simulink model "msdTune"  (R2022b)
settings: Solver=ode23t  StartTime=0.0  StopTime=10  MaxStep=1e-5  RelTol=1e-6
libraries: simulink x2
settings Model: Creator=Rocksmithed  LastModifiedBy=86156
settings SolverCC: AlgebraicLoopSolver=TrustRegion
settings DebuggingCC: UnconnectedInputMsg=warning  UnconnectedOutputMsg=warning  UnconnectedLineMsg=warning  SFMachineParentedDataDiag=warning
settings ModelReferenceCC: EnableRefExpFcnMdlSchedulingChecks=on
settings RTWCC: DLArmComputeVersion=19.05

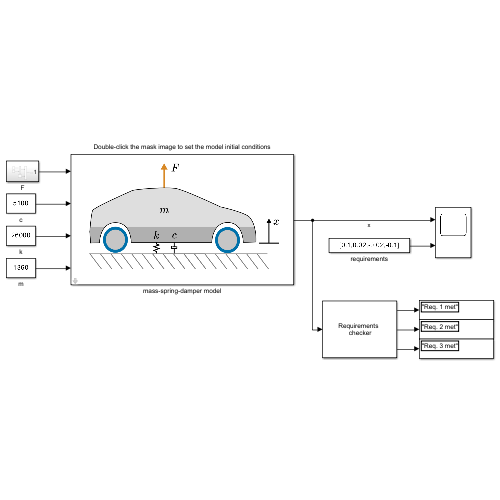
[thumbnail: Simulink's stored preview of the top-level diagram]
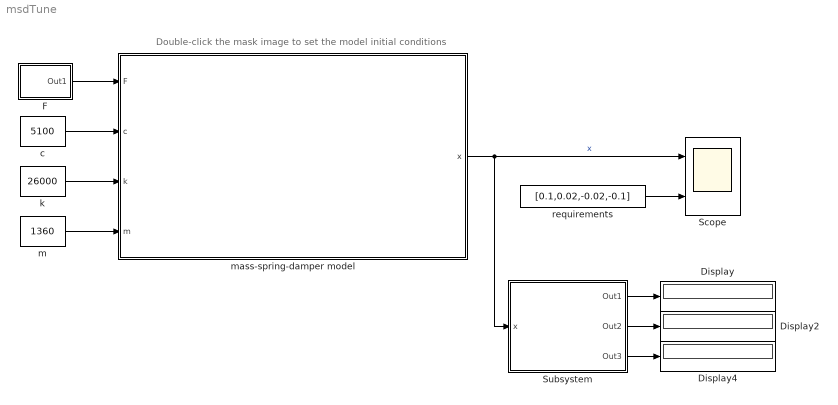
== system msdTune ==
  note: Double-click the mask image to set the model initial conditions
  Display : Display
  Display2 : Display
  Display4 : Display
  F : Subsystem
  Scope : Scope  NumInputPorts=2
  Subsystem : Subsystem
      mask Display: disp('Requirements \n checker')
  c : Constant  Value=5100
  k : Constant  Value=26000
  m : Constant  Value=1360
  mass-spring-damper model : Subsystem  mask{x0=0, x_dot0=0}
      mask prompts: x_dot0 "x'(0)"
      mask Display: image('$imagefile'); % Use "Edit Image" on toolstrip to change.
  requirements : Constant  Value=[0.1,0.02,-0.02,-0.1]
  wires:
  c/1 -> mass-spring-damper model/2(c)
  k/1 -> mass-spring-damper model/3(k)
  m/1 -> mass-spring-damper model/4(m)
  mass-spring-damper model/1(x) -> Subsystem/1(x), Scope/1  "x"
  F/1(Out1) -> mass-spring-damper model/1(F)
  requirements/1 -> Scope/2
  Subsystem/1(Out1) -> Display/1
  Subsystem/2(Out2) -> Display2/1
  Subsystem/3(Out3) -> Display4/1

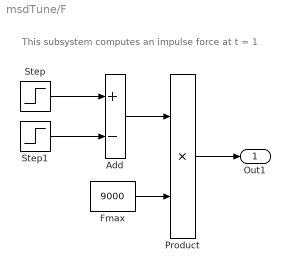
== system msdTune/F ==
  note: This subsystem computes an impulse force at t = 1
  Add : Sum  Inputs=+-
  Fmax : Constant  Value=9000
  Product : Product
  Step : Step  SampleTime=0
  Step1 : Step  Time=1.1  SampleTime=0
  Out1 : Outport
  wires:
  Product/1 -> Out1/1
  Add/1 -> Product/1
  Fmax/1 -> Product/2
  Step/1 -> Add/1
  Step1/1 -> Add/2

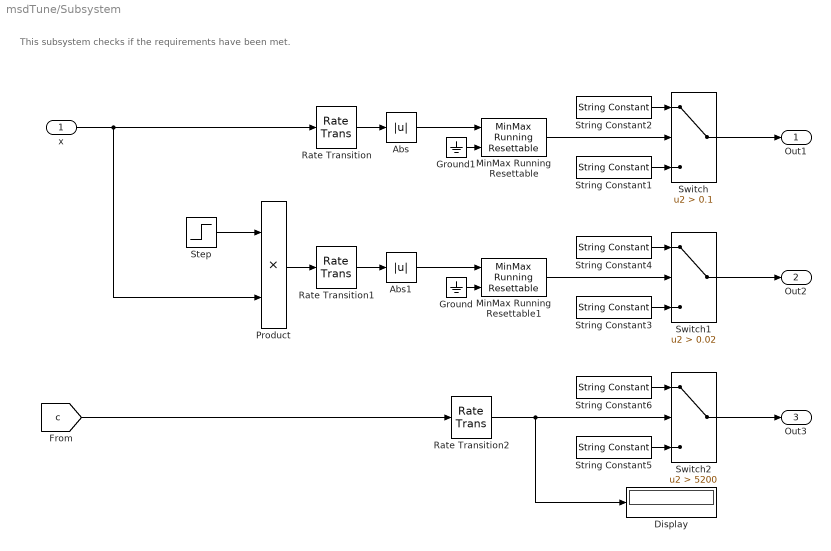
== system msdTune/Subsystem ==
  note: This subsystem checks if the requirements have been met.
  x : Inport
  Abs : Abs  SaturateOnIntegerOverflow=off
  Abs1 : Abs  SaturateOnIntegerOverflow=off
  Display : Display
  Ground : Ground
  Ground1 : Ground
  MinMax Running Resettable : simulink/Math Operations/MinMax Running Resettable  Function=max  vinit=0
  MinMax Running Resettable1 : simulink/Math Operations/MinMax Running Resettable  Function=max  vinit=0
  Product : Product
  Rate Transition : RateTransition  OutPortSampleTime=0.01
  Rate Transition1 : RateTransition  OutPortSampleTime=0.01
  Rate Transition2 : RateTransition  OutPortSampleTime=0.01
  Step : Step  Time=2  SampleTime=0
  String Constant1 : StringConstant  String="\"Req. 1 met\""
  String Constant2 : StringConstant  String="\"Req. 1 not met\""
  String Constant3 : StringConstant  String="\"Req. 2 met\""
  String Constant4 : StringConstant  String="\"Req. 2 not met\""
  String Constant5 : StringConstant  String="\"Req. 3 met\""
  String Constant6 : StringConstant  String="\"Req. 3 not met\""
  Switch : Switch  Criteria=u2 > Threshold  Threshold=0.1  SaturateOnIntegerOverflow=off  InputSameDT=off
  Switch1 : Switch  Criteria=u2 > Threshold  Threshold=0.02  SaturateOnIntegerOverflow=off  InputSameDT=off
  Switch2 : Switch  Criteria=u2 > Threshold  Threshold=5200  SaturateOnIntegerOverflow=off  InputSameDT=off
  Out1 : Outport
  Out2 : Outport  Port=2
  Out3 : Outport  Port=3
  wires:
  [c] -> Rate Transition2/1
  Rate Transition2/1 -> Display/1, Switch2/2
  Step/1 -> Product/1
  MinMax Running Resettable1/1 -> Switch1/2
  String Constant1/1 -> Switch/3
  x/1 -> Product/2, Rate Transition/1
  String Constant2/1 -> Switch/1
  MinMax Running Resettable/1 -> Switch/2
  Abs/1 -> MinMax Running Resettable/1
  Abs1/1 -> MinMax Running Resettable1/1
  Rate Transition1/1 -> Abs1/1
  String Constant4/1 -> Switch1/1
  Switch/1 -> Out1/1
  String Constant3/1 -> Switch1/3
  Product/1 -> Rate Transition1/1
  Rate Transition/1 -> Abs/1
  Switch1/1 -> Out2/1
  Switch2/1 -> Out3/1
  String Constant6/1 -> Switch2/1
  String Constant5/1 -> Switch2/3
  Ground/1 -> MinMax Running Resettable1/2
  Ground1/1 -> MinMax Running Resettable/2

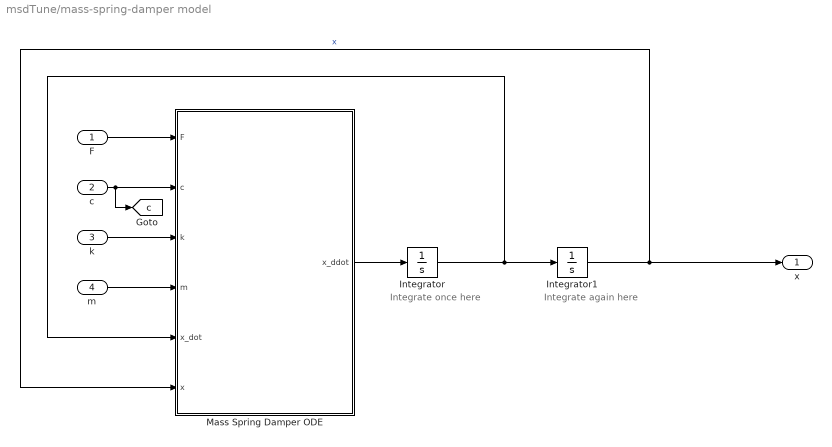
== system msdTune/mass-spring-damper model ==
  note: Integrate once here
  note: Integrate again here
  F : Inport
  c : Inport  Port=2
  k : Inport  Port=3
  m : Inport  Port=4
  Integrator : Integrator  InitialCondition=x_dot0
  Integrator1 : Integrator  InitialCondition=x0
  Mass Spring Damper ODE : MATLAB Function  TreatAsAtomicUnit=on
  x : Outport
  tag scope: c=global
  wires:
  Mass Spring Damper ODE/1(x_ddot) -> Integrator/1
  c/1 -> Mass Spring Damper ODE/2(c), [c]
  Integrator1/1 -> x/1, Mass Spring Damper ODE/6(x)  "x"
  Integrator/1 -> Integrator1/1, Mass Spring Damper ODE/5(x_dot)
  m/1 -> Mass Spring Damper ODE/4(m)
  k/1 -> Mass Spring Damper ODE/3(k)
  F/1 -> Mass Spring Damper ODE/1(F)

== matlab function msdTune/mass-spring-damper model/Mass Spring Damper ODE ==
  data: F input; x_ddot output; c input; k input; m input; x_dot input; x input
function x_ddot = fcn(F,c,k,m,x_dot,x)

   % Write your expression for x_ddot here in terms of the inputs
   x_ddot = -(-F+c.*x_dot+k.*x)./m;
end
